simulink model "H8_2GDL"  (R2022b)
settings: Solver=VariableStepAuto  StartTime=0.0  StopTime=5  RelTol=1e-3
InitFcn:
  | load("hems.mat");
  | airgap = hems.Airgap;
  | current = hems.Current;
  | forceV = hems.Force_Vertical;
  | forceH = hems.Force_Horizontal;
  | inductance = hems.Inductance;
  | resistance = hems.Resistance;
  | 
  | m = 200;
  | g = 9.81;
  | Iyy = 26.887;
  | x_lev12 = 0.443;
  | x_lev34 = 0.542;
  | z_max = 0.0225;
  | z_min = 0.01;
  | z_nom = 0.019375;
  | I_max = 50;
  | I_min = -50;
values from neighbouring files (symbols this model uses):
  Knl = [5091.38390024  -5523.40229407  65.4441805385  -70.1021906971  382.84626499  -986.851041867; -4276.61485995  -4503.65754193  -11.1725652788  -71.2004310761  -295.543801408  -714.324235622]    [Knl.mat]
undefined symbols (not defined in the file or in its folder): hems, lev_nom, magnitude, suelo, techo
libraries: spsMeanLib x1
settings Model: Creator=USUARIO  LastModifiedBy=USUARIO
settings SolverCC: ZeroCrossAlgorithm=Adaptive
settings DebuggingCC: IgnoredZcDiagnostic=none

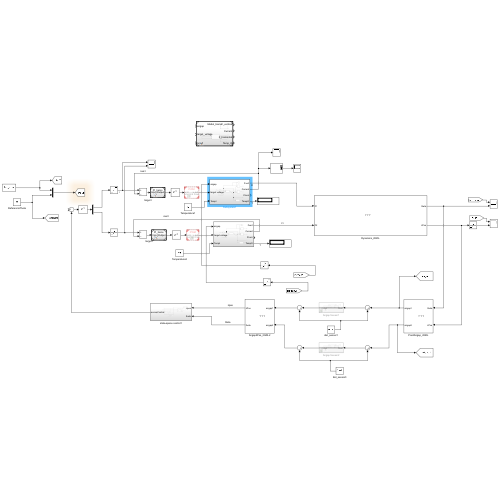
[thumbnail: Simulink's stored preview of the top-level diagram]
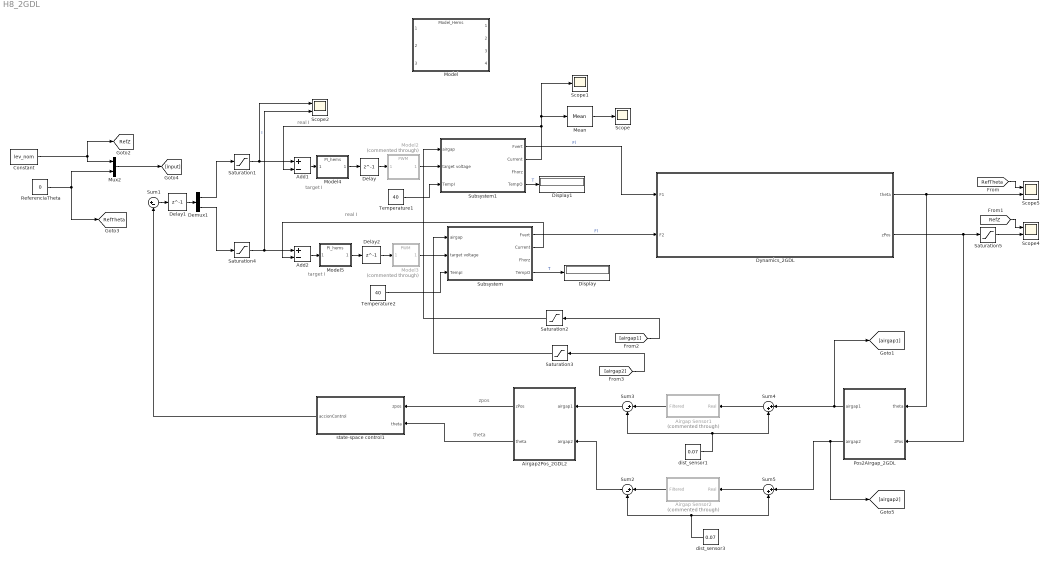
== system H8_2GDL ==
  note: zpos
  note: theta
  note: real I
  note: target I
  note: target I
  note: real I
  Add1 : Sum  Inputs=+-
  Add2 : Sum  Inputs=+-
  Airgap Sensor1 : Subsystem  Commented=through
  Airgap Sensor2 : Subsystem  Commented=through
  Airgap2Pos_2GDL2 : Subsystem
      mask Display: image('C:\Users\ramuj\Desktop\Hyperloop\H8\Levitation-Repository\Levitation-Control-Dynamics\Modelo H8\image_airgapSensor.png'); % Use "Edit Image" on toolstrip to change.
  Constant : Constant  Value=lev_nom
  Delay : Delay  DelayLength=1  SampleTime=1/(5e3)
  Delay1 : Delay  DelayLength=1  SampleTime=1/(1e3)
  Delay2 : Delay  DelayLength=1  SampleTime=1/(5e3)
  Demux1 : Demux  Outputs=2
  Display : Display
  Display1 : Display
  Dynamics_2GDL : Subsystem
      mask Display: image('C:\Users\ramuj\Desktop\Hyperloop\H8\Levitation-Repository\Levitation-Control-Dynamics\ejes.png'); % Use "Edit Image" on toolstrip to change.
  Mean : spsMeanLib/Mean  Freq=6  Vinit=0  Ts=0
  Model : ModelReference  ModelNameDialog=Model_Hems.slx  SimulationMode=Normal  ModelReferenceVersion=1.25
  Model2 : ModelReference  Commented=through  ModelNameDialog=PWM.slx  SimulationMode=Normal  ModelReferenceVersion=1.5
  Model3 : ModelReference  Commented=through  ModelNameDialog=PWM.slx  SimulationMode=Normal  ModelReferenceVersion=1.5
  Model4 : ModelReference  ModelNameDialog=PI_hems.slx  SimulationMode=Normal  ModelReferenceVersion=1.5
  Model5 : ModelReference  ModelNameDialog=PI_hems.slx  SimulationMode=Normal  ModelReferenceVersion=1.5
  Mux2 : Mux  Inputs=2
  Pos2Airgap_2GDL : Subsystem
      mask Display: image('C:\Users\ramuj\Desktop\Hyperloop\H8\Levitation-Repository\Levitation-Control-Dynamics\Modelo H8\image_airgapSensor.png'); % Use "Edit Image" on toolstrip to change.
  ReferenciaTheta : Constant  Value=0
  Saturation1 : Saturate  UpperLimit=I_max  LowerLimit=I_min
  Saturation2 : Saturate  UpperLimit=suelo  LowerLimit=techo
  Saturation3 : Saturate  UpperLimit=suelo  LowerLimit=techo
  Saturation4 : Saturate  UpperLimit=I_max  LowerLimit=I_min
  Saturation5 : Saturate  UpperLimit=suelo  LowerLimit=techo
  Scope : Scope
  Scope1 : Scope
  Scope2 : Scope  NumInputPorts=2
  Scope4 : Scope  NumInputPorts=2
  Scope5 : Scope  NumInputPorts=2
  Subsystem : Subsystem
  Subsystem1 : Subsystem
  Sum1 : Sum  Inputs=|+-
  Sum2 : Sum  Inputs=|+-
  Sum3 : Sum  Inputs=|+-
  Sum4 : Sum  Inputs=|++
  Sum5 : Sum  Inputs=|++
  Temperature1 : Constant  Value=40
  Temperature2 : Constant  Value=40
  dist_sensor1 : Constant  Value=0.07
  dist_sensor3 : Constant  Value=0.07
  state-space control1 : Subsystem
  tag scope: RefTheta=global, RefZ=global
  wires:
  Subsystem1/2(Current) -> Scope1/1, Mean/1, Add1/2
  Subsystem/2(Current) -> Add2/2
  Temperature2/1 -> Subsystem/3(TempI)
  Temperature1/1 -> Subsystem1/3(TempI)
  Dynamics_2GDL/1(theta) -> Pos2Airgap_2GDL/1(theta), Scope5/2
  Dynamics_2GDL/2(zPos) -> Pos2Airgap_2GDL/2(zPos), Saturation5/1
  Subsystem1/1(Fvert) -> Dynamics_2GDL/1(F1)  "Fl"
  Subsystem/1(Fvert) -> Dynamics_2GDL/2(F2)  "Fl"
  Demux1/1 -> Saturation1/1
  Demux1/2 -> Saturation4/1
  Sum1/1 -> Delay1/1
  state-space control1/1(accionControl) -> Sum1/2
  Saturation1/1 -> Scope2/1, Add1/1  "I"
  Add1/1 -> Model4/1
  Model4/1 -> Delay/1
  Saturation4/1 -> Scope2/2, Add2/1
  Add2/1 -> Model5/1
  [RefTheta] -> Scope5/1
  [RefZ] -> Scope4/1
  Saturation2/1 -> Subsystem1/1(airgap)
  Saturation3/1 -> Subsystem/1(airgap)
  Constant/1 -> [RefZ], Mux2/1
  ReferenciaTheta/1 -> Mux2/2, [RefTheta]
  Mux2/1 -> [input]
  Subsystem/4(TempO) -> Display/1  "T"
  Subsystem1/4(TempO) -> Display1/1  "T"
  Sum2/1 -> Airgap2Pos_2GDL2/2(airgap2)
  Sum4/1 -> Airgap Sensor1/1(Real)
  dist_sensor1/1 -> Sum4/2, Sum3/2
  Sum5/1 -> Airgap Sensor2/1(Real)
  Airgap Sensor2/1(Filtered) -> Sum2/1
  Sum3/1 -> Airgap2Pos_2GDL2/1(airgap1)
  Pos2Airgap_2GDL/2(airgap2) -> [airgap2], Sum5/1
  dist_sensor3/1 -> Sum5/2, Sum2/2
  Airgap Sensor1/1(Filtered) -> Sum3/1
  Pos2Airgap_2GDL/1(airgap1) -> [airgap1], Sum4/1
  Airgap2Pos_2GDL2/1(zPos) -> state-space control1/1(zpos)
  Airgap2Pos_2GDL2/2(theta) -> state-space control1/2(theta)
  [airgap1] -> Saturation2/1
  [airgap2] -> Saturation3/1
  Delay1/1 -> Demux1/1
  Delay/1 -> Model2/1
  Delay2/1 -> Model3/1
  Saturation5/1 -> Scope4/2
  Mean/1 -> Scope/1
  Model2/1 -> Subsystem1/2(target voltage)
  Model3/1 -> Subsystem/2(target voltage)
  Model5/1 -> Delay2/1

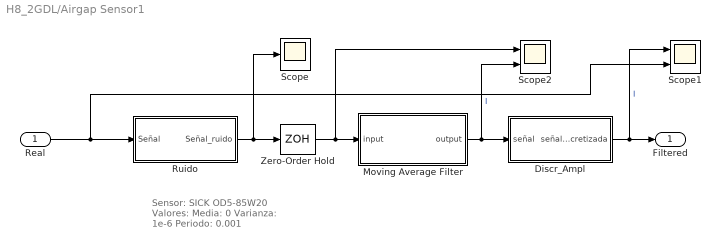
== system H8_2GDL/Airgap Sensor1 ==
  note: Sensor:
      | SICK OD5-85W20
      | Valores:
      | Media: 0
      | Varianza: 1e-6
      | Periodo: 0.001
  Real : Inport
  Discr_Ampl : Subsystem  mask{N=1024, Min=0.065, Max=0.105}
      mask prompts: N "Valores distintos (N)"; Min "Valor mínimo"; Max "Valor máximo"
      mask DialogControl DescGroupVar Prompt: Discretizacion_Amplitud
      mask DialogControl DescTextVar Prompt: Discretización en amplitud
  Moving Average Filter : Subsystem  mask{M=4, fs=-1}
      mask prompts: M "Orden del filtro (M)"; fs "Frecuencia de muestreo (fs)"
  Ruido : Subsystem  mask{M=0, V=1e-7, T=0.001}
      mask prompts: M "Media"; V "Varianza"; T "Periodo"
      mask DialogControl Ruido Prompt: Ruido
      mask DialogControl DescTextVar Prompt: Añade ruido gaussiano
  Scope : Scope
  Scope1 : Scope  NumInputPorts=2
  Scope2 : Scope  NumInputPorts=2
  Zero-Order Hold : ZeroOrderHold  SampleTime=1/(1*10^3)
  Filtered : Outport
  wires:
  Real/1 -> Scope1/2, Ruido/1(Señal)
  Discr_Ampl/1(señal_discretizada) -> Scope1/1, Filtered/1  "I"
  Moving Average Filter/1(output) -> Scope2/2, Discr_Ampl/1(señal)  "I"
  Ruido/1(Señal_ruido) -> Scope/1, Zero-Order Hold/1
  Zero-Order Hold/1 -> Moving Average Filter/1(input), Scope2/1

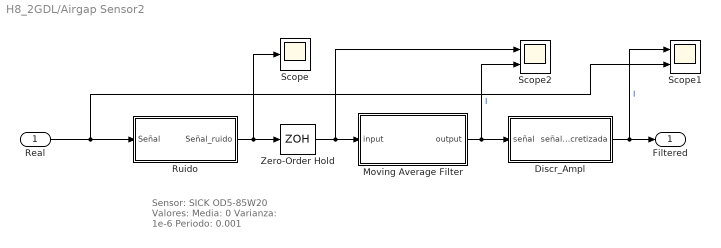
== system H8_2GDL/Airgap Sensor2 ==
  note: Sensor:
      | SICK OD5-85W20
      | Valores:
      | Media: 0
      | Varianza: 1e-6
      | Periodo: 0.001
  Real : Inport
  Discr_Ampl : Subsystem  mask{N=1024, Min=0.065, Max=0.105}
      mask prompts: N "Valores distintos (N)"; Min "Valor mínimo"; Max "Valor máximo"
      mask DialogControl DescGroupVar Prompt: Discretizacion_Amplitud
      mask DialogControl DescTextVar Prompt: Discretización en amplitud
  Moving Average Filter : Subsystem  mask{M=4, fs=-1}
      mask prompts: M "Orden del filtro (M)"; fs "Frecuencia de muestreo (fs)"
  Ruido : Subsystem  mask{M=0, V=1e-7, T=0.001}
      mask prompts: M "Media"; V "Varianza"; T "Periodo"
      mask DialogControl Ruido Prompt: Ruido
      mask DialogControl DescTextVar Prompt: Añade ruido gaussiano
  Scope : Scope
  Scope1 : Scope  NumInputPorts=2
  Scope2 : Scope  NumInputPorts=2
  Zero-Order Hold : ZeroOrderHold  SampleTime=1/(1*10^3)
  Filtered : Outport
  wires:
  Real/1 -> Scope1/2, Ruido/1(Señal)
  Discr_Ampl/1(señal_discretizada) -> Scope1/1, Filtered/1  "I"
  Moving Average Filter/1(output) -> Scope2/2, Discr_Ampl/1(señal)  "I"
  Ruido/1(Señal_ruido) -> Scope/1, Zero-Order Hold/1
  Zero-Order Hold/1 -> Moving Average Filter/1(input), Scope2/1

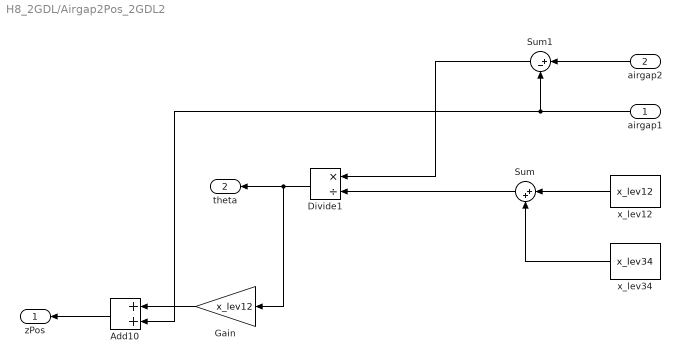
== system H8_2GDL/Airgap2Pos_2GDL2 ==
  airgap1 : Inport
  airgap2 : Inport  Port=2
  Add10 : Sum
  Divide1 : Product  Inputs=*/
  Gain : Gain  Gain=x_lev12
  Sum : Sum  Inputs=|++
  Sum1 : Sum  Inputs=|+-
  x_lev12 : Constant  Value=x_lev12
  x_lev34 : Constant  Value=x_lev34
  zPos : Outport
  theta : Outport  Port=2
  wires:
  Add10/1 -> zPos/1
  Divide1/1 -> theta/1, Gain/1
  x_lev12/1 -> Sum/1
  x_lev34/1 -> Sum/2
  Sum/1 -> Divide1/2
  airgap2/1 -> Sum1/1
  airgap1/1 -> Sum1/2, Add10/2
  Sum1/1 -> Divide1/1
  Gain/1 -> Add10/1

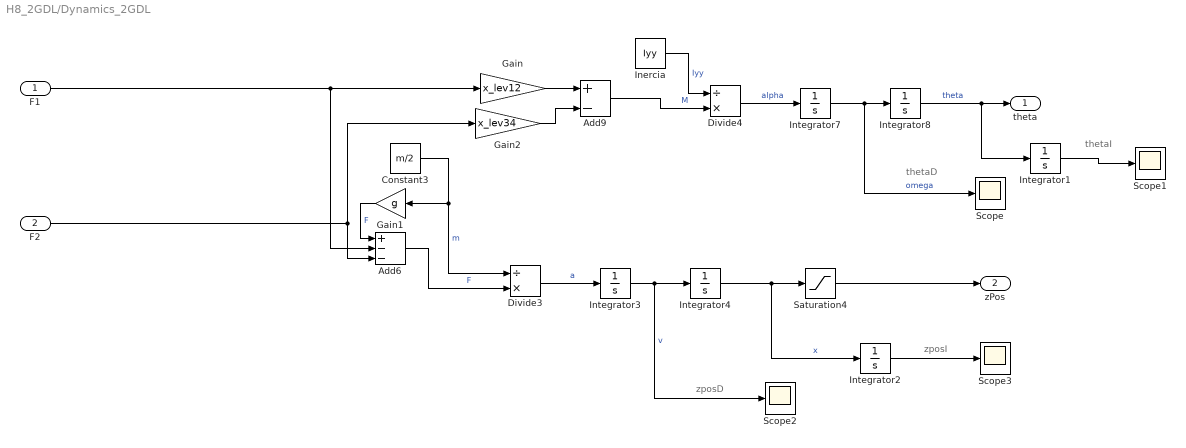
== system H8_2GDL/Dynamics_2GDL ==
  note: thetaI
  note: thetaD
  note: zposD
  note: zposI
  F1 : Inport
  F2 : Inport  Port=2
  Add6 : Sum  Inputs=+--
  Add9 : Sum  Inputs=+-
  Constant3 : Constant  Value=m/2
  Divide3 : Product  Inputs=/*
  Divide4 : Product  Inputs=/*
  Gain : Gain  Gain=x_lev12
  Gain1 : Gain  Gain=g
  Gain2 : Gain  Gain=x_lev34
  Inercia : Constant  Value=Iyy
  Integrator{1,3,7..8} (4 alike) : Integrator
  Integrator2 : Integrator  InitialCondition=suelo  LimitOutput=on  UpperSaturationLimit=suelo  LowerSaturationLimit=techo
  Integrator4 : Integrator  InitialCondition=suelo  LimitOutput=on  UpperSaturationLimit=suelo  LowerSaturationLimit=techo
  Saturation4 : Saturate  UpperLimit=z_max  LowerLimit=z_min
  Scope{,1..3} (4 alike) : Scope
  theta : Outport
  zPos : Outport  Port=2
  wires:
  Saturation4/1 -> zPos/1
  Add6/1 -> Divide3/2  "F"
  Gain/1 -> Add9/1
  Integrator3/1 -> Integrator4/1, Scope2/1  "v"
  F2/1 -> Add6/3, Gain2/1
  Add9/1 -> Divide4/2  "M"
  Integrator4/1 -> Integrator2/1, Saturation4/1  "x"
  Divide3/1 -> Integrator3/1  "a"
  Constant3/1 -> Gain1/1, Divide3/1  "m"
  Inercia/1 -> Divide4/1  "Iyy"
  Integrator8/1 -> Integrator1/1, theta/1  "theta"
  Divide4/1 -> Integrator7/1  "alpha"
  F1/1 -> Gain/1, Add6/2
  Integrator7/1 -> Scope/1, Integrator8/1  "omega"
  Gain1/1 -> Add6/1  "F"
  Gain2/1 -> Add9/2
  Integrator1/1 -> Scope1/1
  Integrator2/1 -> Scope3/1

== system H8_2GDL/Pos2Airgap_2GDL ==
  theta : Inport
  zPos : Inport  Port=2
  Add10 : Sum
  Add11 : Sum  Inputs=-+
  Gain3 : Gain  Gain=x_lev12
  Gain4 : Gain  Gain=x_lev34
  airgap1 : Outport
  airgap2 : Outport  Port=2
  wires:
  Add10/1 -> airgap2/1
  zPos/1 -> Add11/2, Add10/2
  theta/1 -> Gain4/1, Gain3/1
  Gain3/1 -> Add11/1
  Gain4/1 -> Add10/1
  Add11/1 -> airgap1/1

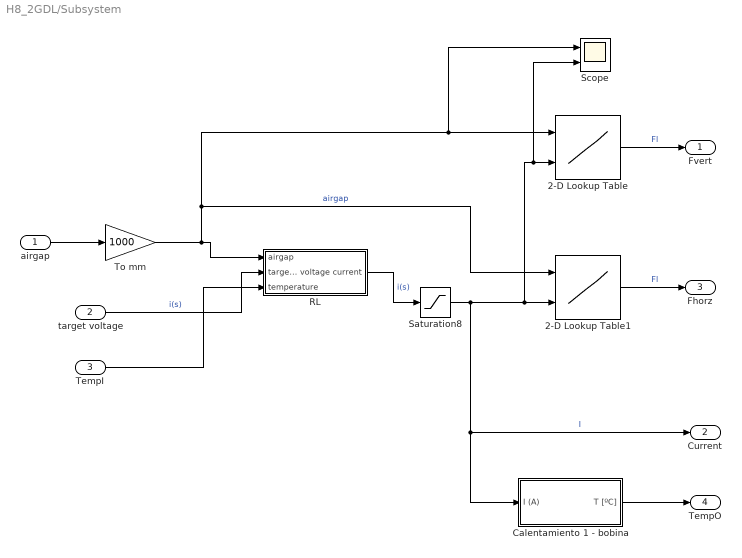
== system H8_2GDL/Subsystem ==
  airgap : Inport
  target voltage : Inport  Port=2
  TempI : Inport  Port=3
  2-D Lookup Table : Lookup_n-D  BreakpointsForDimension1=hems.Airgap'  BreakpointsForDimension2=hems.Current  Table=hems.Force_Vertical  InternalRulePriority=Speed  RndMeth=Simplest
      settings: InputPortMap=u0,u1
  2-D Lookup Table1 : Lookup_n-D  BreakpointsForDimension1=hems.Airgap'  BreakpointsForDimension2=hems.Current  Table=hems.Force_Horizontal  InternalRulePriority=Speed  RndMeth=Simplest
      settings: InputPortMap=u0,u1
  Calentamiento 1 - bobina : Subsystem
  RL : Subsystem
  Saturation8 : Saturate  UpperLimit=50  LowerLimit=-50
  Scope : Scope  NumInputPorts=2
  To mm : Gain  Gain=1000
  Fvert : Outport
  Current : Outport  Port=2
  Fhorz : Outport  Port=3
  TempO : Outport  Port=4
  wires:
  RL/1(current) -> Saturation8/1  "i(s)"
  target voltage/1 -> RL/2(target voltage)  "i(s)"
  To mm/1 -> Scope/1, 2-D Lookup Table/1, 2-D Lookup Table1/1, RL/1(airgap)  "airgap"
  Calentamiento 1 - bobina/1(T [ºC]) -> TempO/1
  2-D Lookup Table1/1 -> Fhorz/1  "Fl"
  Saturation8/1 -> Calentamiento 1 - bobina/1(I (A)), Current/1, 2-D Lookup Table1/2, Scope/2, 2-D Lookup Table/2  "I"
  TempI/1 -> RL/3(temperature)
  airgap/1 -> To mm/1
  2-D Lookup Table/1 -> Fvert/1  "Fl"

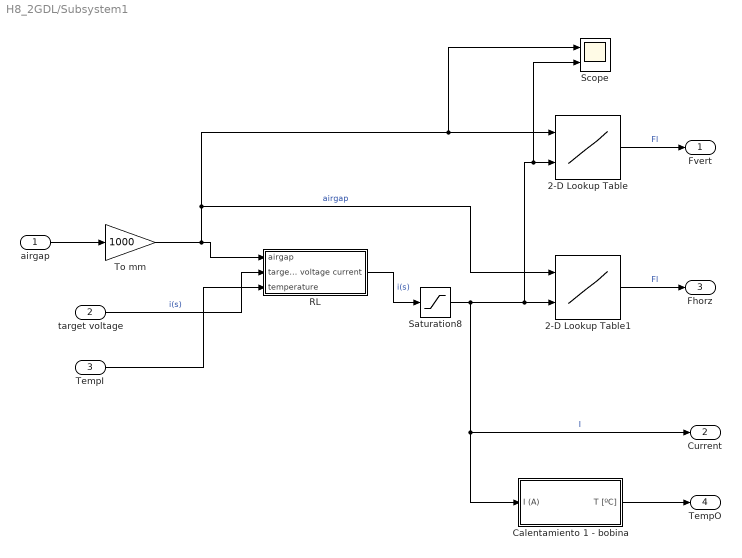
== system H8_2GDL/Subsystem1 ==
  airgap : Inport
  target voltage : Inport  Port=2
  TempI : Inport  Port=3
  2-D Lookup Table : Lookup_n-D  BreakpointsForDimension1=hems.Airgap'  BreakpointsForDimension2=hems.Current  Table=hems.Force_Vertical  InternalRulePriority=Speed  RndMeth=Simplest
      settings: InputPortMap=u0,u1
  2-D Lookup Table1 : Lookup_n-D  BreakpointsForDimension1=hems.Airgap'  BreakpointsForDimension2=hems.Current  Table=hems.Force_Horizontal  InternalRulePriority=Speed  RndMeth=Simplest
      settings: InputPortMap=u0,u1
  Calentamiento 1 - bobina : Subsystem
  RL : Subsystem
  Saturation8 : Saturate  UpperLimit=50  LowerLimit=-50
  Scope : Scope  NumInputPorts=2
  To mm : Gain  Gain=1000
  Fvert : Outport
  Current : Outport  Port=2
  Fhorz : Outport  Port=3
  TempO : Outport  Port=4
  wires:
  RL/1(current) -> Saturation8/1  "i(s)"
  target voltage/1 -> RL/2(target voltage)  "i(s)"
  To mm/1 -> Scope/1, 2-D Lookup Table/1, 2-D Lookup Table1/1, RL/1(airgap)  "airgap"
  Calentamiento 1 - bobina/1(T [ºC]) -> TempO/1
  2-D Lookup Table1/1 -> Fhorz/1  "Fl"
  Saturation8/1 -> Calentamiento 1 - bobina/1(I (A)), Current/1, 2-D Lookup Table1/2, Scope/2, 2-D Lookup Table/2  "I"
  TempI/1 -> RL/3(temperature)
  airgap/1 -> To mm/1
  2-D Lookup Table/1 -> Fvert/1  "Fl"

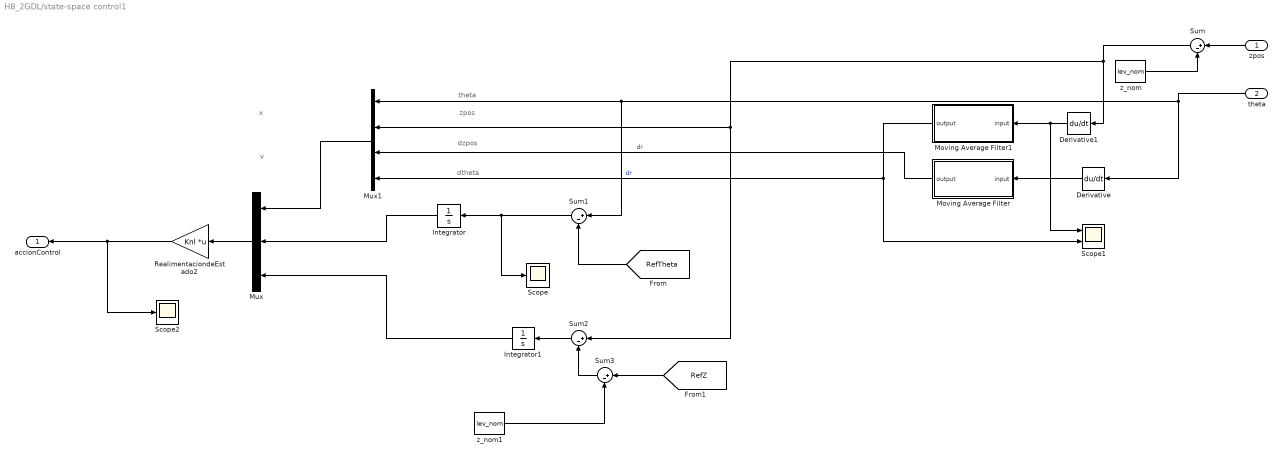
== system H8_2GDL/state-space control1 ==
  note: v
  note: x
  note: dtheta
  note: dzpos
  note: zpos
  note: theta
  zpos : Inport
  theta : Inport  Port=2
  Derivative : Derivative
  Derivative1 : Derivative
  Integrator : Integrator
  Integrator1 : Integrator
  Moving Average Filter : Subsystem  mask{M=4, fs=-1}
      mask prompts: M "Orden del filtro (M)"; fs "Frecuencia de muestreo (fs)"
  Moving Average Filter1 : Subsystem  mask{M=4, fs=-1}
      mask prompts: M "Orden del filtro (M)"; fs "Frecuencia de muestreo (fs)"
  Mux : Mux  Inputs=3
  Mux1 : Mux
  RealimentaciondeEstado2 : Gain  Gain=Knl  Multiplication=Matrix(K*u)
  Scope : Scope
  Scope1 : Scope  NumInputPorts=2
  Scope2 : Scope
  Sum{,1..3} (4 alike) : Sum  Inputs=|+-
  z_nom : Constant  Value=lev_nom
  z_nom1 : Constant  Value=lev_nom
  accionControl : Outport
  wires:
  Derivative1/1 -> Scope1/1, Moving Average Filter1/1(input)
  Mux1/1 -> Mux/1
  theta/1 -> Derivative/1, Sum1/1, Mux1/1
  Derivative/1 -> Moving Average Filter/1(input)
  RealimentaciondeEstado2/1 -> Scope2/1, accionControl/1
  Moving Average Filter/1(output) -> Mux1/3  "dr"
  Moving Average Filter1/1(output) -> Scope1/2, Mux1/4  "dr"
  z_nom/1 -> Sum/2
  zpos/1 -> Sum/1
  Mux/1 -> RealimentaciondeEstado2/1
  Integrator/1 -> Mux/2
  [RefTheta] -> Sum1/2
  Sum1/1 -> Scope/1, Integrator/1
  Sum2/1 -> Integrator1/1
  Sum/1 -> Mux1/2, Sum2/1, Derivative1/1
  Integrator1/1 -> Mux/3
  z_nom1/1 -> Sum3/2
  [RefZ] -> Sum3/1
  Sum3/1 -> Sum2/2

== system H8_2GDL/Airgap Sensor1/Discr_Ampl ==
  señal : Inport
  Constant : Constant  Value=N
  Constant1 : Constant  Value=Max
  Constant2 : Constant  Value=Min
  MATLAB Function1 : MATLAB Function  TreatAsAtomicUnit=on
  señal_discretizada : Outport
  wires:
  MATLAB Function1/1(senal_discretizada) -> señal_discretizada/1
  señal/1 -> MATLAB Function1/1(senal)
  Constant1/1 -> MATLAB Function1/3(Max)
  Constant/1 -> MATLAB Function1/2(N)
  Constant2/1 -> MATLAB Function1/4(Min)

== system H8_2GDL/Airgap Sensor1/Moving Average Filter ==
  input : Inport
  Delay : Delay  DelayLength=M  SampleTime=fs
  Delay1 : Delay  DelayLength=1  SampleTime=fs
  Gain : Gain  Gain=1/M
  Sum : Sum  Inputs=|+-
  Sum1 : Sum  Inputs=|++
  output : Outport
  wires:
  input/1 -> Delay/1, Sum/1
  Delay/1 -> Sum/2
  Sum/1 -> Sum1/1
  Sum1/1 -> Delay1/1, Gain/1
  Delay1/1 -> Sum1/2
  Gain/1 -> output/1

== system H8_2GDL/Airgap Sensor1/Ruido ==
  Señal : Inport
  Random Number : RandomNumber  Mean=M  Variance=V  Seed=3  SampleTime=T
  Sum : Sum  Inputs=|++
  Señal_ruido : Outport
  wires:
  Random Number/1 -> Sum/2
  Señal/1 -> Sum/1
  Sum/1 -> Señal_ruido/1

== system H8_2GDL/Airgap Sensor2/Discr_Ampl ==
  señal : Inport
  Constant : Constant  Value=N
  Constant1 : Constant  Value=Max
  Constant2 : Constant  Value=Min
  MATLAB Function1 : MATLAB Function  TreatAsAtomicUnit=on
  señal_discretizada : Outport
  wires:
  MATLAB Function1/1(senal_discretizada) -> señal_discretizada/1
  señal/1 -> MATLAB Function1/1(senal)
  Constant1/1 -> MATLAB Function1/3(Max)
  Constant/1 -> MATLAB Function1/2(N)
  Constant2/1 -> MATLAB Function1/4(Min)

== system H8_2GDL/Airgap Sensor2/Moving Average Filter ==
  input : Inport
  Delay : Delay  DelayLength=M  SampleTime=fs
  Delay1 : Delay  DelayLength=1  SampleTime=fs
  Gain : Gain  Gain=1/M
  Sum : Sum  Inputs=|+-
  Sum1 : Sum  Inputs=|++
  output : Outport
  wires:
  input/1 -> Delay/1, Sum/1
  Delay/1 -> Sum/2
  Sum/1 -> Sum1/1
  Sum1/1 -> Delay1/1, Gain/1
  Delay1/1 -> Sum1/2
  Gain/1 -> output/1

== system H8_2GDL/Airgap Sensor2/Ruido ==
  Señal : Inport
  Random Number : RandomNumber  Mean=M  Variance=V  Seed=3  SampleTime=T
  Sum : Sum  Inputs=|++
  Señal_ruido : Outport
  wires:
  Random Number/1 -> Sum/2
  Señal/1 -> Sum/1
  Sum/1 -> Señal_ruido/1

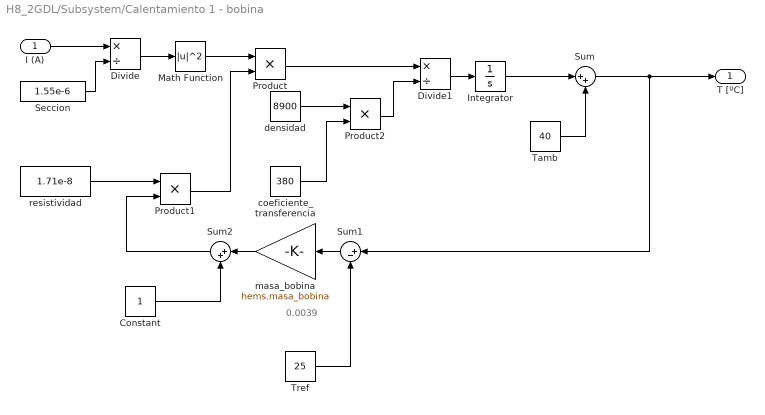
== system H8_2GDL/Subsystem/Calentamiento 1 - bobina ==
  note: 0.0039
  I (A) : Inport
  Constant : Constant
  Divide : Product  Inputs=*/
  Divide1 : Product  Inputs=*/
  Integrator : Integrator
  Math Function : Math  Operator=magnitude^2
  Product : Product
  Product1 : Product
  Product2 : Product
  Seccion : Constant  Value=1.55e-6
  Sum : Sum  Inputs=|++
  Sum1 : Sum  Inputs=|+-
  Sum2 : Sum  Inputs=|++
  Tamb : Constant  Value=40
  Tref : Constant  Value=25
  coeficiente_transferencia : Constant  Value=380
  densidad : Constant  Value=8900
  masa_bobina : Gain  Gain=hems.masa_bobina
  resistividad : Constant  Value=1.71e-8
  T [ºC] : Outport
  wires:
  I (A)/1 -> Divide/1
  Seccion/1 -> Divide/2
  Divide/1 -> Math Function/1
  Math Function/1 -> Product/1
  Product/1 -> Divide1/1
  Divide1/1 -> Integrator/1
  Integrator/1 -> Sum/1
  Tamb/1 -> Sum/2
  Sum/1 -> Sum1/1, T [ºC]/1
  Sum1/1 -> masa_bobina/1
  Tref/1 -> Sum1/2
  masa_bobina/1 -> Sum2/1
  Constant/1 -> Sum2/2
  resistividad/1 -> Product1/1
  Sum2/1 -> Product1/2
  Product1/1 -> Product/2
  Product2/1 -> Divide1/2
  densidad/1 -> Product2/1
  coeficiente_transferencia/1 -> Product2/2

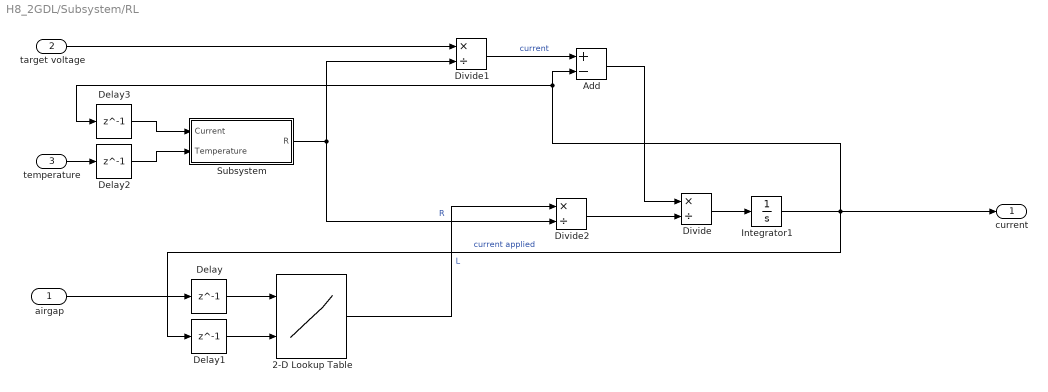
== system H8_2GDL/Subsystem/RL ==
  airgap : Inport
  target voltage : Inport  Port=2
  temperature : Inport  Port=3
  2-D Lookup Table : Lookup_n-D  BreakpointsForDimension1=hems.Airgap  BreakpointsForDimension2=hems.Current(2:110)  Table=hems.Inductance  InternalRulePriority=Speed  RndMeth=Simplest
      settings: InputPortMap=u0,u1
  Add : Sum  Inputs=+-
  Delay{,1..3} (4 alike) : Delay  DelayLength=1
  Divide : Product  Inputs=*/
  Divide1 : Product  Inputs=*/
  Divide2 : Product  Inputs=*/
  Integrator1 : Integrator
  Subsystem : Subsystem
  current : Outport
  wires:
  airgap/1 -> Delay/1
  Divide/1 -> Integrator1/1
  Add/1 -> Divide/1
  Integrator1/1 -> Delay1/1, current/1, Delay3/1, Add/2  "current applied"
  2-D Lookup Table/1 -> Divide2/1  "L"
  target voltage/1 -> Divide1/1
  temperature/1 -> Delay2/1
  Divide1/1 -> Add/1  "current"
  Subsystem/1(R) -> Divide2/2, Divide1/2  "R"
  Delay3/1 -> Subsystem/1(Current)
  Delay2/1 -> Subsystem/2(Temperature)
  Divide2/1 -> Divide/2
  Delay1/1 -> 2-D Lookup Table/2
  Delay/1 -> 2-D Lookup Table/1

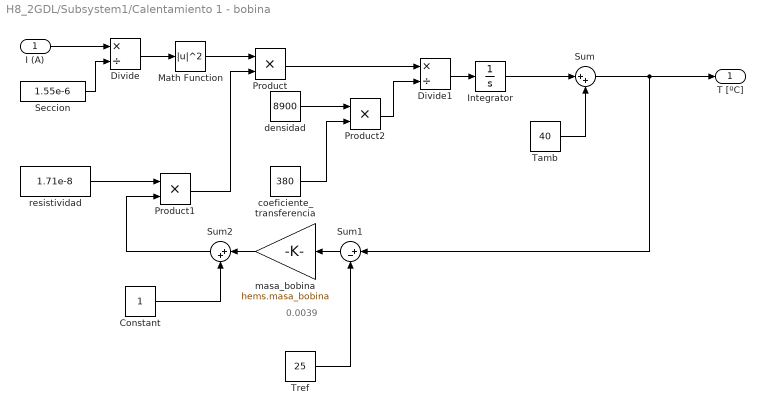
== system H8_2GDL/Subsystem1/Calentamiento 1 - bobina ==
  note: 0.0039
  I (A) : Inport
  Constant : Constant
  Divide : Product  Inputs=*/
  Divide1 : Product  Inputs=*/
  Integrator : Integrator
  Math Function : Math  Operator=magnitude^2
  Product : Product
  Product1 : Product
  Product2 : Product
  Seccion : Constant  Value=1.55e-6
  Sum : Sum  Inputs=|++
  Sum1 : Sum  Inputs=|+-
  Sum2 : Sum  Inputs=|++
  Tamb : Constant  Value=40
  Tref : Constant  Value=25
  coeficiente_transferencia : Constant  Value=380
  densidad : Constant  Value=8900
  masa_bobina : Gain  Gain=hems.masa_bobina
  resistividad : Constant  Value=1.71e-8
  T [ºC] : Outport
  wires:
  I (A)/1 -> Divide/1
  Seccion/1 -> Divide/2
  Divide/1 -> Math Function/1
  Math Function/1 -> Product/1
  Product/1 -> Divide1/1
  Divide1/1 -> Integrator/1
  Integrator/1 -> Sum/1
  Tamb/1 -> Sum/2
  Sum/1 -> Sum1/1, T [ºC]/1
  Sum1/1 -> masa_bobina/1
  Tref/1 -> Sum1/2
  masa_bobina/1 -> Sum2/1
  Constant/1 -> Sum2/2
  resistividad/1 -> Product1/1
  Sum2/1 -> Product1/2
  Product1/1 -> Product/2
  Product2/1 -> Divide1/2
  densidad/1 -> Product2/1
  coeficiente_transferencia/1 -> Product2/2

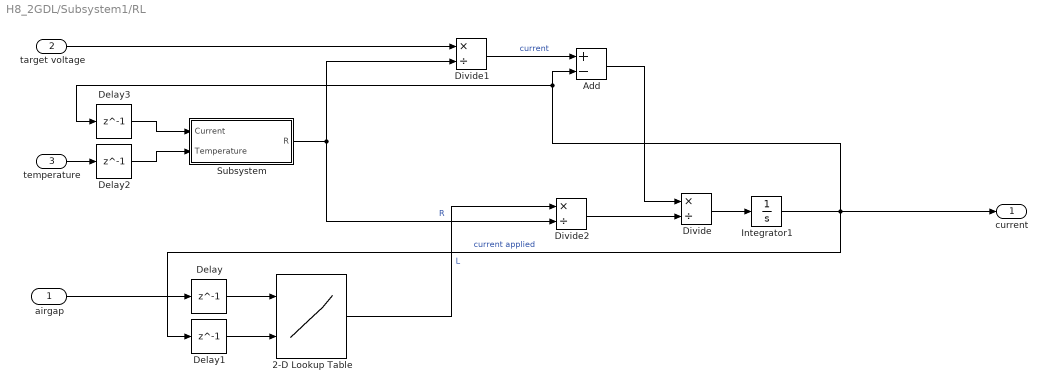
== system H8_2GDL/Subsystem1/RL ==
  airgap : Inport
  target voltage : Inport  Port=2
  temperature : Inport  Port=3
  2-D Lookup Table : Lookup_n-D  BreakpointsForDimension1=hems.Airgap  BreakpointsForDimension2=hems.Current(2:110)  Table=hems.Inductance  InternalRulePriority=Speed  RndMeth=Simplest
      settings: InputPortMap=u0,u1
  Add : Sum  Inputs=+-
  Delay{,1..3} (4 alike) : Delay  DelayLength=1
  Divide : Product  Inputs=*/
  Divide1 : Product  Inputs=*/
  Divide2 : Product  Inputs=*/
  Integrator1 : Integrator
  Subsystem : Subsystem
  current : Outport
  wires:
  airgap/1 -> Delay/1
  Divide/1 -> Integrator1/1
  Add/1 -> Divide/1
  Integrator1/1 -> Delay1/1, current/1, Delay3/1, Add/2  "current applied"
  2-D Lookup Table/1 -> Divide2/1  "L"
  target voltage/1 -> Divide1/1
  temperature/1 -> Delay2/1
  Divide1/1 -> Add/1  "current"
  Subsystem/1(R) -> Divide2/2, Divide1/2  "R"
  Delay3/1 -> Subsystem/1(Current)
  Delay2/1 -> Subsystem/2(Temperature)
  Divide2/1 -> Divide/2
  Delay1/1 -> 2-D Lookup Table/2
  Delay/1 -> 2-D Lookup Table/1

== system H8_2GDL/state-space control1/Moving Average Filter ==
  input : Inport
  Delay : Delay  DelayLength=M  SampleTime=fs
  Delay1 : Delay  DelayLength=1  SampleTime=fs
  Gain : Gain  Gain=1/M
  Sum : Sum  Inputs=|+-
  Sum1 : Sum  Inputs=|++
  output : Outport
  wires:
  input/1 -> Delay/1, Sum/1
  Delay/1 -> Sum/2
  Sum/1 -> Sum1/1
  Sum1/1 -> Delay1/1, Gain/1
  Delay1/1 -> Sum1/2
  Gain/1 -> output/1

== system H8_2GDL/state-space control1/Moving Average Filter1 ==
  input : Inport
  Delay : Delay  DelayLength=M  SampleTime=fs
  Delay1 : Delay  DelayLength=1  SampleTime=fs
  Gain : Gain  Gain=1/M
  Sum : Sum  Inputs=|+-
  Sum1 : Sum  Inputs=|++
  output : Outport
  wires:
  input/1 -> Delay/1, Sum/1
  Delay/1 -> Sum/2
  Sum/1 -> Sum1/1
  Sum1/1 -> Delay1/1, Gain/1
  Delay1/1 -> Sum1/2
  Gain/1 -> output/1

== system H8_2GDL/Subsystem/RL/Subsystem ==
  Current : Inport
  Temperature : Inport  Port=2
  Resistance : Constant  Value=hems.Resistance
  R : Outport
  wires:
  Resistance/1 -> R/1

== system H8_2GDL/Subsystem1/RL/Subsystem ==
  Current : Inport
  Temperature : Inport  Port=2
  Resistance : Constant  Value=hems.Resistance
  R : Outport
  wires:
  Resistance/1 -> R/1

== matlab function H8_2GDL/Airgap Sensor1/Discr_Ampl/MATLAB Function1 ==
  data: senal input; senal_discretizada output; N input; Max input; Min input
function senal_discretizada  = fcn(senal,N,Max,Min)

if(senal>Max)
    senal_discretizada=Max;
    return
elseif(senal<Min)
    senal_discretizada=Min;
    return
end

valor_escalon=(Max-Min)/(N-1);
i=Min;
 while(i<Max)
    if(i+valor_escalon/2>senal)
        senal_discretizada=i;
        return
    end
    i=i+valor_escalon;
end

      senal_discretizada=Max;
end

== matlab function H8_2GDL/Airgap Sensor2/Discr_Ampl/MATLAB Function1 ==
  data: senal input; senal_discretizada output; N input; Max input; Min input
function senal_discretizada  = fcn(senal,N,Max,Min)

if(senal>Max)
    senal_discretizada=Max;
    return
elseif(senal<Min)
    senal_discretizada=Min;
    return
end

valor_escalon=(Max-Min)/(N-1);
i=Min;
 while(i<Max)
    if(i+valor_escalon/2>senal)
        senal_discretizada=i;
        return
    end
    i=i+valor_escalon;
end

      senal_discretizada=Max;
end
